simulink model "time_delay_discrete_model"  (R2023b)
settings: Solver=VariableStepAuto  StartTime=0.0  StopTime=30  RelTol=1e-3
undefined symbols (not defined in the file): A, AAd, Ad, Adtilde, Aimp, B, Bd, Bdtilde, Bimp, C, Cd, Cdtilde, Cimp, D, Ddtilde, Dimp, ei, Ko, nutildei, t_d, xi
settings Model: Creator=tamas  LastModifiedBy=tamas

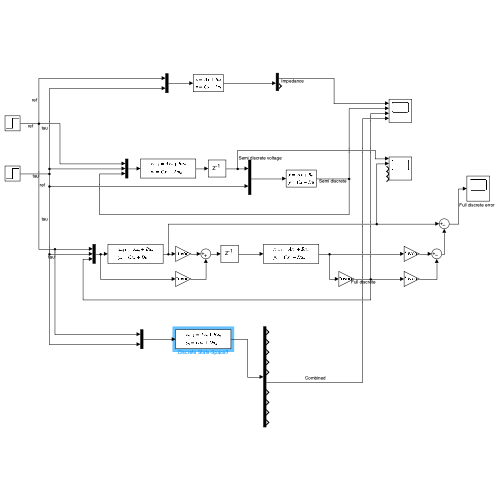
[thumbnail: Simulink's stored preview of the top-level diagram]
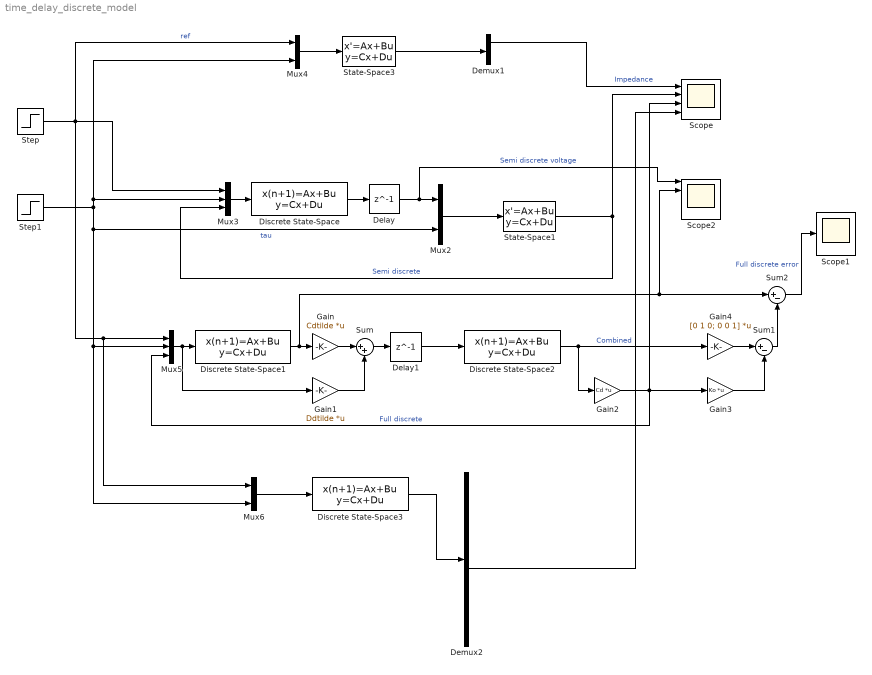
== system time_delay_discrete_model ==
  Delay : Delay  DelayLength=1  InitialCondition=0
  Delay1 : Delay  DelayLength=1  InitialCondition=0
  Demux1 : Demux  Outputs=2
  Demux2 : Demux  Outputs=10
  Discrete State-Space : DiscreteStateSpace  A=Adtilde  B=Bdtilde  C=Cdtilde  D=Ddtilde  InitialCondition=nutildei  SampleTime=t_d
  Discrete State-Space1 : DiscreteStateSpace  A=Adtilde  B=Bdtilde  C=eye(2)  D=zeros([2, 3])  InitialCondition=nutildei  SampleTime=t_d
  Discrete State-Space2 : DiscreteStateSpace  A=Ad  B=Bd  C=eye(3)  D=zeros([3, 1])  InitialCondition=xi  SampleTime=t_d
  Discrete State-Space3 : DiscreteStateSpace  A=AAd  B=zeros([10, 2])  C=eye(10)  D=zeros([10, 2])  InitialCondition=[zeros(5, 1); xi; ei]  SampleTime=t_d
  Gain : Gain  Gain=Cdtilde  Multiplication=Matrix(K*u) (u vector)
  Gain1 : Gain  Gain=Ddtilde  Multiplication=Matrix(K*u) (u vector)
  Gain2 : Gain  Gain=Cd  Multiplication=Matrix(K*u) (u vector)
  Gain3 : Gain  Gain=Ko  Multiplication=Matrix(K*u) (u vector)
  Gain4 : Gain  Gain=[0 1 0; 0 0 1]  Multiplication=Matrix(K*u) (u vector)
  Mux2 : Mux  Inputs=2
  Mux3 : Mux  Inputs=3
  Mux4 : Mux  Inputs=2
  Mux5 : Mux  Inputs=3
  Mux6 : Mux  Inputs=2
  Scope : Scope  NumInputPorts=4
  Scope1 : Scope
  Scope2 : Scope  NumInputPorts=5
  State-Space1 : StateSpace  A=A  B=B  C=C  D=D  InitialCondition=xi
  State-Space3 : StateSpace  A=Aimp  B=Bimp  C=Cimp  D=Dimp  InitialCondition=xi(1:2)
  Step : Step  Time=0  After=0  SampleTime=0
  Step1 : Step  Time=0  After=0  SampleTime=0
  Sum : Sum  Inputs=|++
  Sum1 : Sum  Inputs=|+-
  Sum2 : Sum  Inputs=|+-
  wires:
  State-Space1/1 -> Scope/2, Mux3/3  "Semi discrete"
  Mux2/1 -> State-Space1/1
  Mux3/1 -> Discrete State-Space/1
  Mux4/1 -> State-Space3/1
  State-Space3/1 -> Demux1/1
  Delay/1 -> Scope2/1, Mux2/1  "Semi discrete voltage"
  Discrete State-Space/1 -> Delay/1
  Demux1/1 -> Scope/1  "Impedance"
  Discrete State-Space2/1 -> Gain2/1, Gain4/1
  Step/1 -> Mux6/1, Mux5/1, Mux3/1, Mux4/1  "ref"
  Step1/1 -> Mux5/2, Mux6/2, Mux2/2, Mux3/2, Mux4/2  "tau"
  Delay1/1 -> Discrete State-Space2/1
  Mux5/1 -> Gain1/1, Discrete State-Space1/1
  Discrete State-Space1/1 -> Scope2/2, Sum2/1, Gain/1
  Demux2/6 -> Scope/4  "Combined"
  Gain/1 -> Sum/1
  Sum/1 -> Delay1/1
  Gain1/1 -> Sum/2
  Gain2/1 -> Scope/3, Gain3/1, Mux5/3  "Full discrete"
  Gain4/1 -> Sum1/1
  Gain3/1 -> Sum1/2
  Sum1/1 -> Sum2/2
  Sum2/1 -> Scope1/1  "Full discrete error"
  Mux6/1 -> Discrete State-Space3/1
  Discrete State-Space3/1 -> Demux2/1
